simulink model "LinearizzazioneFeedback_rev4"  (R2024b)
settings: Solver=VariableStepAuto  StartTime=0.0  StopTime=30  FixedStep=0.016  RelTol=2.84e-14
values from neighbouring files (symbols this model uses):
  K = acker(A, b, p)    [main_FeedbLinear.m]
settings Model: Creator=alexi  LastModifiedBy=aldos
settings SolverCC: MaxConsecutiveMinStep=auto  ZeroCrossControl=DisableAll
settings OptimizationCC: ReuseModelBlockBuffer=off
settings RTWCC: GPUComputeCapability=3.5

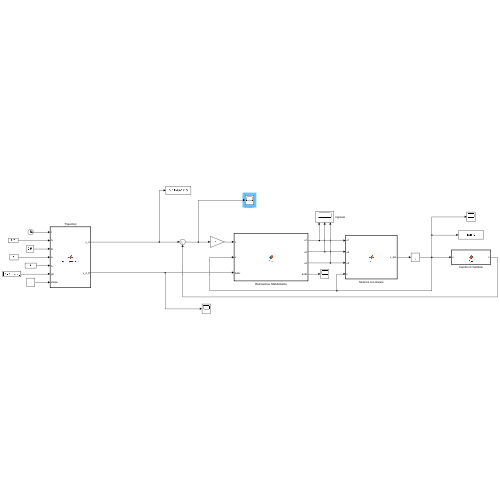
[thumbnail: Simulink's stored preview of the top-level diagram]
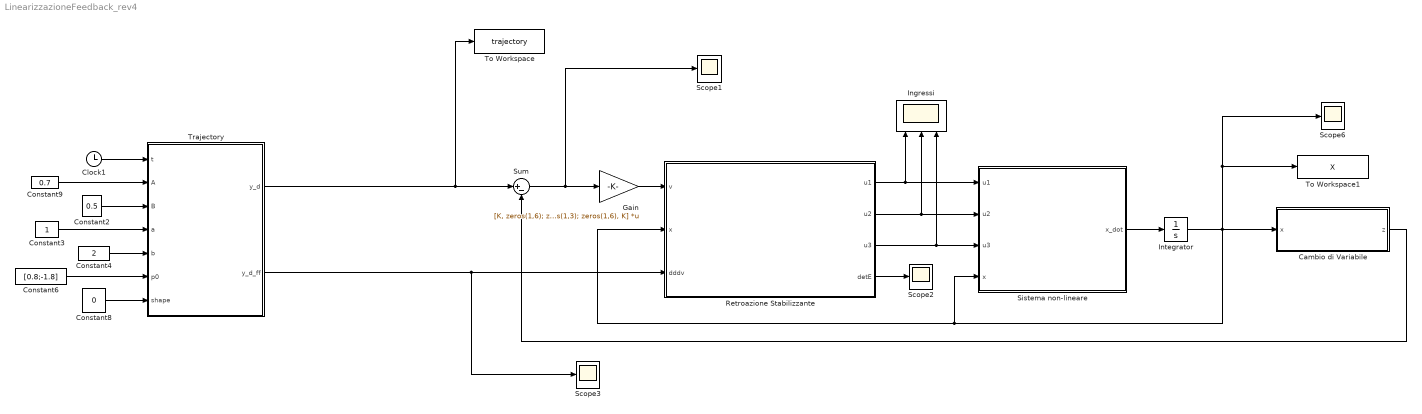
== system LinearizzazioneFeedback_rev4 ==
  " Trajectory" : MATLAB Function  TreatAsAtomicUnit=on
  Cambio di Variabile : MATLAB Function  TreatAsAtomicUnit=on
  Clock1 : Clock
      settings: Decimation=30
  Constant2 : Constant  Value=0.5
  Constant3 : Constant
  Constant4 : Constant  Value=2
  Constant6 : Constant  Value=[0.8;-1.8]
  Constant8 : Constant  Value=0
  Constant9 : Constant  Value=0.7
  Gain : Gain  Gain=[K, zeros(1,6); zeros(1,3), K, zeros(1,3); zeros(1,6), K]  Multiplication=Matrix(K*u)
  Ingressi : Scope  NumInputPorts=3
  Integrator : Integrator  InitialCondition=[0.2 0.2 0.2 0.0 0.0 0.0 0.2 0.2 0.2]'
  Retroazione Stabilizzante : MATLAB Function  TreatAsAtomicUnit=on
  Scope{1..3,6} (4 alike) : Scope
  Sistema non-lineare : MATLAB Function  TreatAsAtomicUnit=on
  Sum : Sum  Inputs=|+-
  To Workspace : ToWorkspace  VariableName=trajectory  SaveFormat=Timeseries  SampleTime=-1
  To Workspace1 : ToWorkspace  VariableName=X  SaveFormat=Timeseries  SampleTime=-1
  wires:
  Integrator/1 -> To Workspace1/1, Scope6/1, Sistema non-lineare/4(x), Retroazione Stabilizzante/2(x), Cambio di Variabile/1(x)
  Retroazione Stabilizzante/1(u1) -> Sistema non-lineare/1(u1), Ingressi/1
  Retroazione Stabilizzante/2(u2) -> Sistema non-lineare/2(u2), Ingressi/2
  " Trajectory"/1(y_d) -> To Workspace/1, Sum/1
  Retroazione Stabilizzante/3(u3) -> Sistema non-lineare/3(u3), Ingressi/3
  Retroazione Stabilizzante/4(detE) -> Scope2/1
  Sistema non-lineare/1(x_dot) -> Integrator/1
  Clock1/1 -> " Trajectory"/1(t)
  Constant3/1 -> " Trajectory"/4(a)
  Constant9/1 -> " Trajectory"/2(A)
  Constant4/1 -> " Trajectory"/5(b)
  Constant6/1 -> " Trajectory"/6(p0)
  Constant2/1 -> " Trajectory"/3(B)
  Constant8/1 -> " Trajectory"/7(shape)
  Cambio di Variabile/1(z) -> Sum/2
  Sum/1 -> Gain/1, Scope1/1
  Gain/1 -> Retroazione Stabilizzante/1(v)
  " Trajectory"/2(y_d_ff) -> Scope3/1, Retroazione Stabilizzante/3(dddv)

== matlab function LinearizzazioneFeedback_rev4/Cambio di Variabile ==
  data: x input; z output
function z = fcn(x)
a1 = 1;
a2 = 1;
a3 = 1;
k1 = 15; k2 = 15; k3 = 15;      % rigidezze molle
q1 = x(1);
q2 = x(2);
q3 = x(3);
dq1 = x(4);
dq2 = x(5);
dq3 = x(6);
theta1 = x(7);
theta2 = x(8);
theta3 = x(9);


B = RR_mass_matrix(q1,q2,q3);
C = RR_coriolis_matrix(q1,q2,q3,dq1,dq2,dq3);
G = RR_gravity_vector(q1,q2,q3);


inversa_b = inv(B);

b1_1 = inversa_b(1,1);
b1_2 = inversa_b(1,2);
b1_3 = inversa_b(1,3);
b2_1 = inversa_b(2,1);
b2_2 = inversa_b(2,2);
b2_3 = inversa_b(2,3);
b3_1 = inversa_b(3,1);
b3_2 = inversa_b(3,2);
b3_3 = inversa_b(3,3);


c1_1 = C(1,1);
c1_2 = C(1,2);
c1_3 = C(1,3);
c2_1 = C(2,1);
c2_2 = C(2,2);
c2_3 = C(2,3);
c3_1 = C(3,1);
c3_2 = C(3,2);
c3_3 = C(3,3);

g1 = G(1);
g2 = G(2);
g3 = G(3);


z1 = a1*cos(q1)+a2*cos(q1+q2)+a3*cos(q1+q2+q3); %posizione in x
z2 = -a1*sin(q1)*dq1 -a2*sin(q1+q2)*(dq1+dq2) - a3*sin(q1+q2+q3)*(dq1+dq2+dq3); %derivata prima
z3 = sin(q1)*(b1_1*g1 + b1_2*g2 + b1_3*g3 + dq1*(b1_1*c1_1 + b1_2*c2_1 + b1_3*c3_1) + dq2*(b1_1*c1_2 + b1_2*c2_2 + b1_3*c3_2) + dq3*(b1_1*c1_3 + b1_2*c2_3 + b1_3*c3_3) + b1_1*k1*(q1 - theta1) + b1_2*k2*(q2 - theta2) + b1_3*k3*(q3 - theta3)) - cos(q1 + q2 + q3)*(dq1 + dq2 + dq3)^2 - cos(q1 + q2)*(dq1 + dq2)^2 + sin(q1 + q2)*(b1_1*g1 + b1_2*g2 + b1_3*g3 + b2_1*g1 + b2_2*g2 + b2_3*g3 + dq1*(b1_1*c1_1 + b1_2*c2_1 + b1_3*c3_1) + dq2*(b1_1*c1_2 + b1_2*c2_2 + b1_3*c3_2) + dq3*(b1_1*c1_3 + b1_2*c2_3 + b1_3*c3_3) + dq1*(b2_1*c1_1 + b2_2*c2_1 + b2_3*c3_1) + dq2*(b2_1*c1_2 + b2_2*c2_2 + b2_3*c3_2) + dq3*(b2_1*c1_3 + b2_2*c2_3 + b2_3*c3_3) + b1_1*k1*(q1 - theta1) + b1_2*k2*(q2 - theta2) + b1_3*k3*(q3 - theta3) + b2_1*k1*(q1 - theta1) + b2_2*k2*(q2 - theta2) + b2_3*k3*(q3 - theta3)) + sin(q1 + q2 + q3)*(b1_1*g1 + b1_2*g2 + b1_3*g3 + b2_1*g1 + b2_2*g2 + b2_3*g3 + b3_1*g1 + b3_2*g2 + b3_3*g3 + dq1*(b1_1*c1_1 + b1_2*c2_1 + b1_3*c3_1) + dq2*(b1_1*c1_2 + b1_2*c2_2 + b1_3*c3_2) + dq3*(b1_1*c1_3 + b1_2*c2_3 + b1_3*c3_3) + dq1*(b2_1*c1_1 + b2_2*c2_1 + b2_3*c3_1) + dq2*(b2_1*c1_2 + b2_2*c2_2 + b2_3*c3_2) + dq3*(b2_1*c1_3 + b2_2*c2_3 + b2_3*c3_3) + dq1*(b3_1*c1_1 + b3_2*c2_1 + b3_3*c3_1) + dq2*(b3_1*c1_2 + b3_2*c2_2 + b3_3*c3_2) + dq3*(b3_1*c1_3 + b3_2*c2_3 + b3_3*c3_3) + b1_1*k1*(q1 - theta1) + b1_2*k2*(q2 - theta2) + b1_3*k3*(q3 - theta3) + b2_1*k1*(q1 - theta1) + b2_2*k2*(q2 - theta2) + b2_3*k3*(q3 - theta3) + b3_1*k1*(q1 - theta1) + b3_2*k2*(q2 - theta2) + b3_3*k3*(q3 - theta3)) - dq1^2*cos(q1);


z4 =    a1*sin(q1)+a2*sin(q1+q2)+a3*sin(q1+q2+q3); %posizione in y
z5 =    a1*cos(q1)*dq1 + a2*cos(q1+q2)*(dq1+dq2) + a3*cos(q1+q2+q3)*(dq1+dq2+dq3);
z6 =   - dq1^2*sin(q1) - cos(q1)*(b1_1*g1 + b1_2*g2 + b1_3*g3 + dq1*(b1_1*c1_1 + b1_2*c2_1 + b1_3*c3_1) + dq2*(b1_1*c1_2 + b1_2*c2_2 + b1_3*c3_2) + dq3*(b1_1*c1_3 + b1_2*c2_3 + b1_3*c3_3) + b1_1*k1*(q1 - theta1) + b1_2*k2*(q2 - theta2) + b1_3*k3*(q3 - theta3)) - sin(q1 + q2 + q3)*(dq1 + dq2 + dq3)^2 - sin(q1 + q2)*(dq1 + dq2)^2 - cos(q1 + q2)*(b1_1*g1 + b1_2*g2 + b1_3*g3 + b2_1*g1 + b2_2*g2 + b2_3*g3 + dq1*(b1_1*c1_1 + b1_2*c2_1 + b1_3*c3_1) + dq2*(b1_1*c1_2 + b1_2*c2_2 + b1_3*c3_2) + dq3*(b1_1*c1_3 + b1_2*c2_3 + b1_3*c3_3) + dq1*(b2_1*c1_1 + b2_2*c2_1 + b2_3*c3_1) + dq2*(b2_1*c1_2 + b2_2*c2_2 + b2_3*c3_2) + dq3*(b2_1*c1_3 + b2_2*c2_3 + b2_3*c3_3) + b1_1*k1*(q1 - theta1) + b1_2*k2*(q2 - theta2) + b1_3*k3*(q3 - theta3) + b2_1*k1*(q1 - theta1) + b2_2*k2*(q2 - theta2) + b2_3*k3*(q3 - theta3)) - cos(q1 + q2 + q3)*(b1_1*g1 + b1_2*g2 + b1_3*g3 + b2_1*g1 + b2_2*g2 + b2_3*g3 + b3_1*g1 + b3_2*g2 + b3_3*g3 + dq1*(b1_1*c1_1 + b1_2*c2_1 + b1_3*c3_1) + dq2*(b1_1*c1_2 + b1_2*c2_2 + b1_3*c3_2) + dq3*(b1_1*c1_3 + b1_2*c2_3 + b1_3*c3_3) + dq1*(b2_1*c1_1 + b2_2*c2_1 + b2_3*c3_1) + dq2*(b2_1*c1_2 + b2_2*c2_2 + b2_3*c3_2) + dq3*(b2_1*c1_3 + b2_2*c2_3 + b2_3*c3_3) + dq1*(b3_1*c1_1 + b3_2*c2_1 + b3_3*c3_1) + dq2*(b3_1*c1_2 + b3_2*c2_2 + b3_3*c3_2) + dq3*(b3_1*c1_3 + b3_2*c2_3 + b3_3*c3_3) + b1_1*k1*(q1 - theta1) + b1_2*k2*(q2 - theta2) + b1_3*k3*(q3 - theta3) + b2_1*k1*(q1 - theta1) + b2_2*k2*(q2 - theta2) + b2_3*k3*(q3 - theta3) + b3_1*k1*(q1 - theta1) + b3_2*k2*(q2 - theta2) + b3_3*k3*(q3 - theta3));

z7 = q3;
z8 = dq3;
z9 =- b3_1*g1 - b3_2*g2 - b3_3*g3 - dq1*(b3_1*c1_1 + b3_2*c2_1 + b3_3*c3_1) - dq2*(b3_1*c1_2 + b3_2*c2_2 + b3_3*c3_2) - dq3*(b3_1*c1_3 + b3_2*c2_3 + b3_3*c3_3) - b3_1*k1*(q1 - theta1) - b3_2*k2*(q2 - theta2) - b3_3*k3*(q3 - theta3);

z = [z1 z2 z3 z4 z5 z6 z7 z8 z9]';

== matlab function LinearizzazioneFeedback_rev4/Retroazione Stabilizzante ==
  data: v input; u1 output; x input; u2 output; dddv input; u3 output; detE output
function [u1, u2, u3, detE]= fcn(v, x, dddv)
v1 = v(1);
v2 = v(2);
v3 = v(3);

k1 = 15; k2 = 15; k3 = 15;   % Rigidezza
q1 = x(1);
q2 = x(2);
q3 = x(3);
dq1 = x(4);
dq2 = x(5);
dq3 = x(6);
theta1 = x(7);
theta2 = x(8);
theta3 = x(9);


E = matE( q1, q2, q3, k1, k2, k3);

F = matgam(q1, q2, q3, dq1, dq2, dq3, ...
          theta1, theta2, theta3, ...
          k1, k2, k3);


detE = det(E);
v = [v1; v2; v3];
o = dddv + v;
% u = -inv(E)*F + inv(E)*o;
% u = - inv(E)*F + E\o;

u =  E\(o - F);

u1 = u(1);
u2 = u(2);
u3 = u(3);

== matlab function LinearizzazioneFeedback_rev4/ Trajectory ==
  data: t input; y_d output; A input; B input; a input; b input; p0 input; shape input; y_d_ff output
function [y_d, y_d_ff]= traj_generator(t, A, B, a, b, p0, shape)
% Traiettoria cartesiana: Lissajous o Circolare
% shape = 0 --> Lissajous
% shape = 1 --> Circonferenza

    if shape == 0
        % ----- Lissajous -----
        xi_des   = [A*sin(a*t); B*sin(b*t)] + p0;
        dxi_des  = [A*a*cos(a*t); B*b*cos(b*t)];
        ddxi_des = [-A*a^2*sin(a*t); -B*b^2*sin(b*t)];
        dddp     = [-A*a^3*cos(a*t); -B*b^3*cos(b*t)];

        q3_amp = pi/3;        % Ampiezza oscillazione (30 gradi)
        q3_freq = 3 * a;    % Frequenza scelta arbitrariamente
        q3     = q3_amp * sin(q3_freq * t);
        dq3    = q3_amp * q3_freq * cos(q3_freq * t);
        ddq3   = -q3_amp * q3_freq^2 * sin(q3_freq * t);
        dddq3  = -q3_amp * q3_freq^3 * cos(q3_freq * t);

    else
        % ----- Circonferenza -----
        % Uso A come raggio, a come velocità angolare
        R = A; 
        omega = a;

        xi_des   = [R*cos(omega*t); R*sin(omega*t)] + p0;
        dxi_des  = [-R*omega*sin(omega*t); R*omega*cos(omega*t)];
        ddxi_des = [-R*omega^2*cos(omega*t); -R*omega^2*sin(omega*t)];
        dddp     = [R*omega^3*sin(omega*t); -R*omega^3*cos(omega*t)];
        
        q3_amp = pi/4;        % Ampiezza oscillazione (30 gradi)
        q3_freq = 3 * a;    % Frequenza scelta arbitrariamente
        q3     = q3_amp * sin(q3_freq * t);
        dq3    = q3_amp * q3_freq * cos(q3_freq * t);
        ddq3   = -q3_amp * q3_freq^2 * sin(q3_freq * t);
        dddq3  = -q3_amp * q3_freq^3 * cos(q3_freq * t);
    end

    y_d = [xi_des(1), dxi_des(1), ddxi_des(1), xi_des(2), dxi_des(2), ddxi_des(2) , q3, dq3, ddq3]';
    y_d_ff = [dddp ; dddq3];
end

== matlab function LinearizzazioneFeedback_rev4/Sistema non-lineare ==
  data: u1 input; x_dot output; u2 input; u3 input; x input
function x_dot   = fcn(u1,u2,u3,x)
%x=[q1 q2 q3 dq1 dq2 dq3 theta1 theta2 theta3]

% ingressi: u1 = dtheta1, u2 = dtheta2  (velocità motori)
%
% Parametri (modifica secondo i tuoi valori)
k1 = 15; k2 = 15; k3 = 15;      % rigidezze molle
% b1 = 2*sqrt(1*k1); b2 = 2*sqrt(1*k2); b3 = 2*sqrt(1*k3);   % smorzamenti viscous (opzionali)
b1 = 0.0; b2 = 0.0; b3 = 0.0;

% estrazione stato
q  = x(1:3);
dq = x(4:6);
theta = x(7:9);

% coppie elastiche + viscose
tau1 = k1*(theta(1) - q(1))+b1*(u1-dq(1));  % tra motore1 e giunto1
tau2 = k2*(theta(2) - q(2))+b2*(u2-dq(2));  % tra motore2 e giunto2
tau3 = k3*(theta(3) - q(3))+b3*(u3-dq(3));  % tra motore3 e giunto2   

tau = [tau1; tau2; tau3];


% DINAMICA: usa le tue funzioni per M, C, G (adattare nomi se diversi)
M = RR_mass_matrix(q(1),q(2),q(3));           % 3x3
C = RR_coriolis_matrix(q(1),q(2),q(3),dq(1),dq(2),dq(3));    % 3x3, tale che C*dq = coriolis term
G = RR_gravity_vector(q(1),q(2),q(3));        % 3x1



% calcolo accelerazioni giunti (numericamente stabile)
ddq = inv(M)*( tau - C*dq - G );

% costruzione derivata di stato
x_dot = zeros(9,1);

x_dot(1:3)   = dq;
x_dot(4:6)   = ddq;
x_dot(7)     = u1;   % theta1_dot = u1
x_dot(8)     = u2;   % theta2_dot = u2
x_dot(9)     = u3;   % theta3_dot = u3
